simulink model "PathFollower"  (R2024b)
settings: Solver=FixedStepAuto  StartTime=0.0  StopTime=inf  FixedStep=controllerParams.Ts  RelTol=1e-3
PreLoadFcn:
  | % Load scenario parameters if not already loaded
  | if ~exist('hostParams', 'var')
  |     hostParams = helperScenarioParams;
  | end
  | 
  | % Load vehicle parameters if not already loaded
  | if ~exist('vehicleParams', 'var')
  |     vehicleParams = helperVehicleParams;
  | end
  | 
  | % Load PathFollower parameters if not already loaded
  | if ~exist('controllerParams', 'var')
  |     controllerParams = helperPathFollowerParams;
  | end
  | 
  | % Set IP addresses to local computer if they are not provided
  | if ~exist('ipAddress', 'var')
  |     ipAddress = helperIPAddresses;
  | end
libraries: slrealtimeiplib x4, slrealtimeutilitieslib x3, slpidlib x2, simulink x2, robotalgslib x1
settings Model: SimulationMode=external  ExtModeBatchMode=on  ExtModeTrigDuration=100000  Creator=smaddina  LastModifiedBy=demo-user2
settings SolverCC: ConcurrentTasks=on  PositivePriorityOrder=on
settings OptimizationCC: BlockReduction=off  OptimizeBlockIOStorage=off  EnhancedBackFolding=on  PassReuseOutputArgsThreshold=0  MaxStackSize=200000  OptimizeBlockOrder=speed  DifferentSizesBufferReuse=on
settings DebuggingCC: TasksWithSamePriorityMsg=none  ParameterTunabilityLossMsg=error
settings HardwareCC: ProdBitPerLong=64  ProdLongLongMode=on  ProdHWDeviceType=Intel->x86-64 (Linux 64)
settings SFSimCC: MATLABDynamicMemAlloc=off
settings RTWCC: Description=Speedgoat Real-Time Target Machine  SystemTargetFile=speedgoat.tlc  TemplateMakefile=slrealtime_default_tmf  Toolchain=Simulink Real-Time Toolchain  BuildConfiguration=Faster Runs  CodeExecutionProfiling=on  TargetLang=C++
settings CodeAppCC: ForceParamTrailComments=on  OperatorAnnotations=on
settings SimulinkRealTimeTargetCC: InstructionSetFMA=off  LogToMDFFile=off

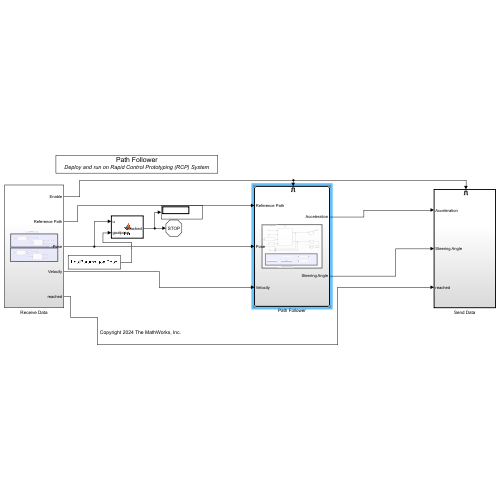
[thumbnail: Simulink's stored preview of the top-level diagram]
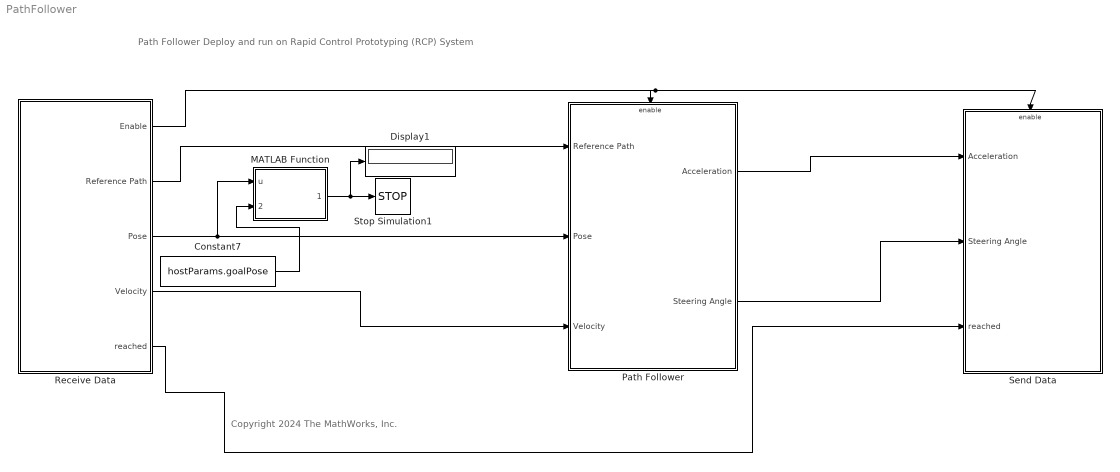
== system PathFollower ==
  note: Path Follower
      | Deploy and run on Rapid Control Prototyping (RCP) System
  note: Copyright 2024 The MathWorks, Inc.
  Constant7 : Constant  Value=hostParams.goalPose
  Display1 : Display
  MATLAB Function : MATLAB Function  TreatAsAtomicUnit=on
  Path Follower : Subsystem
  Receive Data : Subsystem
  Send Data : Subsystem
  Stop Simulation1 : Stop
  wires:
  Receive Data/3(Pose) -> MATLAB Function/1(u), Path Follower/2(Pose)
  Path Follower/1(Acceleration) -> Send Data/1(Acceleration)
  Receive Data/2(Reference Path) -> Path Follower/1(Reference Path)
  Receive Data/4(Velocity) -> Path Follower/3(Velocity)
  Path Follower/2(Steering Angle) -> Send Data/2(Steering Angle)
  Receive Data/1(Enable) -> Send Data/Enable, Path Follower/Enable
  Receive Data/5(reached) -> Send Data/3(reached)
  Constant7/1 -> MATLAB Function/2(goalpose)
  MATLAB Function/1(reached) -> Display1/1, Stop Simulation1/1

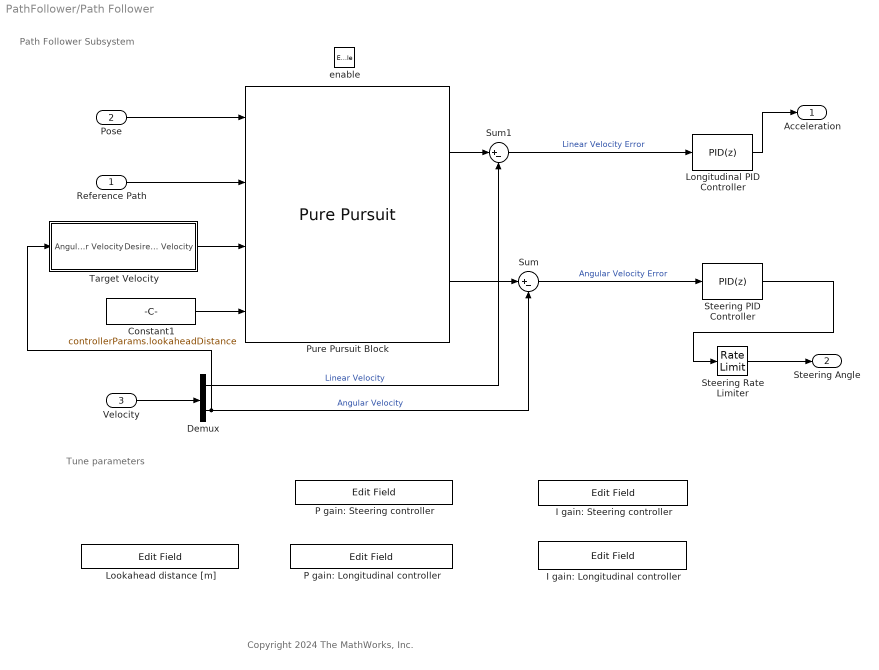
== system PathFollower/Path Follower ==
  note: Path Follower Subsystem
  note: Tune parameters
  note: Copyright 2024 The MathWorks, Inc.
  Reference Path : Inport
  Pose : Inport  Port=2
  Velocity : Inport  Port=3  Interpolate=off
  enable : EnablePort  StatesWhenEnabling=reset
  "       I gain: Longitudinal controller" : EditField  LabelPosition=Hide  ShowInitialText=on  Alignment=Center
  "   I gain: Steering controller" : EditField  LabelPosition=Hide  ShowInitialText=on  Alignment=Center
  Constant1 : Constant  Value=controllerParams.lookaheadDistance
  Demux : Demux  Outputs=2
  Longitudinal PID Controller : slpidlib/PID Controller  Controller=PID  Form=Parallel  TimeDomain=Discrete-time  UseExternalTs=off  SampleTime=-1  IntegratorMethod=Forward Euler  FilterMethod=Forward Euler  ControllerParametersSource=internal  P=controllerParams.accelPGain  I=controllerParams.accelIGain  UseKiTs=off  D=0  UseExternalDerivativeSource=off  N=0  UseFilter=on  TunerSelectOption=Transfer Function Based (PID Tuner App)  InitialConditionSource=internal  InitialConditionForIntegrator=0  InitialConditionForFilter=0  DifferentiatorICPrevScaledInput=0  ExternalReset=none  TrackingMode=off  Kt=1  LimitOutput=on  SatLimitsSource=internal  UpperSaturationLimit=vehicleParams.maxAcceleration  LowerSaturationLimit=vehicleParams.maxDeceleration  LinearizeAsGain=on  AntiWindupMode=none  Kb=1  LimitIntegrator=off  UpperIntegratorSaturationLimit=inf  LowerIntegratorSaturationLimit=-inf  POutMin=[]  POutMax=[]  IOutMin=[]  IOutMax=[]  DOutMin=[]  DOutMax=[]  NOutMin=[]  NOutMax=[]  SumOutMin=[]  SumOutMax=[]  SaturationOutMin=[]  SaturationOutMax=[]  PParamMin=[]  PParamMax=[]  IParamMin=[]  IParamMax=[]  DParamMin=[]  DParamMax=[]  NParamMin=[]  NParamMax=[]  KbParamMin=[]  KbParamMax=[]  KtParamMin=[]  KtParamMax=[]  KbOutMin=[]  KbOutMax=[]  KtOutMin=[]  KtOutMax=[]  IntegratorOutMin=[]  IntegratorOutMax=[]  FilterOutMin=[]  FilterOutMax=[]  SumI1OutMin=[]  SumI1OutMax=[]  SumI2OutMin=[]  SumI2OutMax=[]  SumI3OutMin=[]  SumI3OutMax=[]  SumI4OutMin=[]  SumI4OutMax=[]  SumDOutMin=[]  SumDOutMax=[]  DifferentiatorOutMin=[]  DifferentiatorOutMax=[]  FilterDiffOutCoefMin=[]  FilterDiffOutCoefMax=[]  ReciprocalOutMin=[]  ReciprocalOutMax=[]  SumDenOutMin=[]  SumDenOutMax=[]  SumNumOutMin=[]  SumNumOutMax=[]  DivideOutMin=[]  DivideOutMax=[]  UdiffTsProdOutMin=[]  UdiffTsProdOutMax=[]  NTsProdOutMin=[]  NTsProdOutMax=[]  UintegralTsProdOutMin=[]  UintegralTsProdOutMax=[]  UngainTsProdOutMin=[]  UngainTsProdOutMax=[]  ClampingZeroOutDataTypeStr=Inherit: Inherit via back propagation  ClampingZeroOutMin=[]  ClampingZeroOutMax=[]  FilterDenConstantOutDataTypeStr=Inherit: Inherit via back propagation  FilterDenConstantOutMin=[]  FilterDenConstantOutMax=[]  PCopyOutDataTypeStr=Inherit: Inherit via back propagation  PCopyOutMin=[]  PCopyOutMax=[]  NCopyOutDataTypeStr=Inherit: Inherit via back propagation  NCopyOutMin=[]  NCopyOutMax=[]  IntegratorContinuousStateAttributes=''  IntegratorStateMustResolveToSignalObject=off  IntegratorRTWStateStorageClass=Auto  FilterContinuousStateAttributes=''  FilterStateMustResolveToSignalObject=off  FilterRTWStateStorageClass=Auto  ParallelPVariant=InternalParameters  IdealPVariant=Disabled  IVariant=InternalParameters  DVariant=InternalParameters  IntegratorVariant=Discrete  SatVariant=Enabled  AWVariant=Passthrough  PCopyVariant=Disabled  TRVariant=Disabled  FdbkBlocksVariant=Forward  IdealPFdbkVariant=Disabled  SatFdbkVariant=Disabled  DerivativeFilterVariant=ForwardEulerFilter  NVariant=InternalParameters  NCopyVariant=Disabled  FilterICVariant=InternalICsFilter  IntegratorICVariant=InternalICs  ExternalResetVariant=Disabled  TRSumVariant=Passthrough  SumFdbkVariant=Disabled  SumVariant=Sum_PID  TsampFilterVariant=InternalTs  TsampNgainVariant=Passthrough  TsampIntegralVariant=Disabled_SignalSpec  ExternalSaturationOutDataTypeStr=Inherit: Same as second input  DerivativeSourceVariant=ErrorSignal  PreIntVariant=InternalPreInt
  Lookahead distance [m] : EditField  LabelPosition=Hide  ShowInitialText=on  Alignment=Center
  P gain: Longitudinal controller : EditField  LabelPosition=Hide  ShowInitialText=on  Alignment=Center
  P gain: Steering controller : EditField  LabelPosition=Hide  ShowInitialText=on  Alignment=Center
  Pure Pursuit Block : robotalgslib/Pure Pursuit  DesiredLinearVelocityPort=on  DesiredLinearVelocity=5  MaxAngularVelocity=vehicleParams.maxAngularVelocity  LookaheadDistancePort=on  LookaheadDistance=5  TargetDirPort=off  SimulateUsing=Interpreted execution
  Steering Rate Limiter : RateLimiter  RisingSlewLimit=vehicleParams.maxSteeringAngleRate  FallingSlewLimit=-vehicleParams.maxSteeringAngleRate  SampleTimeMode=inherited
  Steering PID Controller : slpidlib/PID Controller  Controller=PID  Form=Parallel  TimeDomain=Discrete-time  UseExternalTs=off  SampleTime=-1  IntegratorMethod=Forward Euler  FilterMethod=Forward Euler  ControllerParametersSource=internal  P=controllerParams.steeringPGain  I=controllerParams.steeringIGain  UseKiTs=off  D=0  UseExternalDerivativeSource=off  N=0  UseFilter=on  TunerSelectOption=Transfer Function Based (PID Tuner App)  InitialConditionSource=internal  InitialConditionForIntegrator=0  InitialConditionForFilter=0  DifferentiatorICPrevScaledInput=0  ExternalReset=none  TrackingMode=off  Kt=1  LimitOutput=on  SatLimitsSource=internal  UpperSaturationLimit=vehicleParams.maxSteeringAngleRate  LowerSaturationLimit=-vehicleParams.maxSteeringAngleRate  LinearizeAsGain=on  AntiWindupMode=none  Kb=1  LimitIntegrator=off  UpperIntegratorSaturationLimit=inf  LowerIntegratorSaturationLimit=-inf  POutMin=[]  POutMax=[]  IOutMin=[]  IOutMax=[]  DOutMin=[]  DOutMax=[]  NOutMin=[]  NOutMax=[]  SumOutMin=[]  SumOutMax=[]  SaturationOutMin=[]  SaturationOutMax=[]  PParamMin=[]  PParamMax=[]  IParamMin=[]  IParamMax=[]  DParamMin=[]  DParamMax=[]  NParamMin=[]  NParamMax=[]  KbParamMin=[]  KbParamMax=[]  KtParamMin=[]  KtParamMax=[]  KbOutMin=[]  KbOutMax=[]  KtOutMin=[]  KtOutMax=[]  IntegratorOutMin=[]  IntegratorOutMax=[]  FilterOutMin=[]  FilterOutMax=[]  SumI1OutMin=[]  SumI1OutMax=[]  SumI2OutMin=[]  SumI2OutMax=[]  SumI3OutMin=[]  SumI3OutMax=[]  SumI4OutMin=[]  SumI4OutMax=[]  SumDOutMin=[]  SumDOutMax=[]  DifferentiatorOutMin=[]  DifferentiatorOutMax=[]  FilterDiffOutCoefMin=[]  FilterDiffOutCoefMax=[]  ReciprocalOutMin=[]  ReciprocalOutMax=[]  SumDenOutMin=[]  SumDenOutMax=[]  SumNumOutMin=[]  SumNumOutMax=[]  DivideOutMin=[]  DivideOutMax=[]  UdiffTsProdOutMin=[]  UdiffTsProdOutMax=[]  NTsProdOutMin=[]  NTsProdOutMax=[]  UintegralTsProdOutMin=[]  UintegralTsProdOutMax=[]  UngainTsProdOutMin=[]  UngainTsProdOutMax=[]  ClampingZeroOutDataTypeStr=Inherit: Inherit via back propagation  ClampingZeroOutMin=[]  ClampingZeroOutMax=[]  FilterDenConstantOutDataTypeStr=Inherit: Inherit via back propagation  FilterDenConstantOutMin=[]  FilterDenConstantOutMax=[]  PCopyOutDataTypeStr=Inherit: Inherit via back propagation  PCopyOutMin=[]  PCopyOutMax=[]  NCopyOutDataTypeStr=Inherit: Inherit via back propagation  NCopyOutMin=[]  NCopyOutMax=[]  IntegratorContinuousStateAttributes=''  IntegratorStateMustResolveToSignalObject=off  IntegratorRTWStateStorageClass=Auto  FilterContinuousStateAttributes=''  FilterStateMustResolveToSignalObject=off  FilterRTWStateStorageClass=Auto  ParallelPVariant=InternalParameters  IdealPVariant=Disabled  IVariant=InternalParameters  DVariant=InternalParameters  IntegratorVariant=Discrete  SatVariant=Enabled  AWVariant=Passthrough  PCopyVariant=Disabled  TRVariant=Disabled  FdbkBlocksVariant=Forward  IdealPFdbkVariant=Disabled  SatFdbkVariant=Disabled  DerivativeFilterVariant=ForwardEulerFilter  NVariant=InternalParameters  NCopyVariant=Disabled  FilterICVariant=InternalICsFilter  IntegratorICVariant=InternalICs  ExternalResetVariant=Disabled  TRSumVariant=Passthrough  SumFdbkVariant=Disabled  SumVariant=Sum_PID  TsampFilterVariant=InternalTs  TsampNgainVariant=Passthrough  TsampIntegralVariant=Disabled_SignalSpec  ExternalSaturationOutDataTypeStr=Inherit: Same as second input  DerivativeSourceVariant=ErrorSignal  PreIntVariant=InternalPreInt
  Sum : Sum  Inputs=|+-
  Sum1 : Sum  Inputs=|+-
  Target Velocity : Subsystem
  Acceleration : Outport
  Steering Angle : Outport  Port=2
  wires:
  Sum/1 -> Steering PID Controller/1  "Angular Velocity Error"
  Velocity/1 -> Demux/1
  Pure Pursuit Block/2 -> Sum/1
  Reference Path/1 -> Pure Pursuit Block/2
  Pose/1 -> Pure Pursuit Block/1
  Demux/1 -> Sum1/2  "Linear Velocity"
  Demux/2 -> Sum/2, Target Velocity/1(Angular Velocity)  "Angular Velocity"
  Steering Rate Limiter/1 -> Steering Angle/1
  Sum1/1 -> Longitudinal PID Controller/1  "Linear Velocity Error"
  Longitudinal PID Controller/1 -> Acceleration/1
  Pure Pursuit Block/1 -> Sum1/1
  Constant1/1 -> Pure Pursuit Block/4
  Target Velocity/1(Desired Velocity) -> Pure Pursuit Block/3
  Steering PID Controller/1 -> Steering Rate Limiter/1

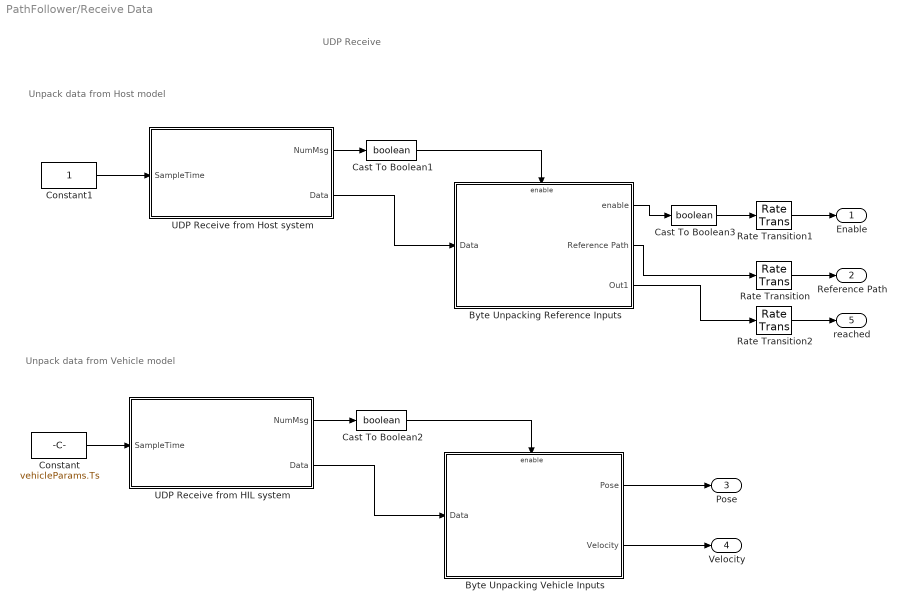
== system PathFollower/Receive Data ==
  note: Unpack data from Vehicle model
  note: Unpack data from Host model
  note: UDP Receive
  Byte Unpacking Reference Inputs : Subsystem  TreatAsAtomicUnit=on
  Byte Unpacking Vehicle Inputs : Subsystem  TreatAsAtomicUnit=on
  Cast To Boolean1 : DataTypeConversion  OutDataTypeStr=boolean  SaturateOnIntegerOverflow=off  RndMeth=Floor
  Cast To Boolean2 : DataTypeConversion  OutDataTypeStr=boolean  SaturateOnIntegerOverflow=off  RndMeth=Floor
  Cast To Boolean3 : DataTypeConversion  OutDataTypeStr=boolean  SaturateOnIntegerOverflow=off  RndMeth=Floor
  Constant : Constant  Value=vehicleParams.Ts  SampleTime=vehicleParams.Ts
  Constant1 : Constant  SampleTime=1
  Rate Transition : RateTransition
  Rate Transition1 : RateTransition
  Rate Transition2 : RateTransition
  UDP Receive from HIL system : Subsystem  TreatAsAtomicUnit=on
  UDP Receive from Host system : Subsystem  TreatAsAtomicUnit=on
  Enable : Outport
  Reference Path : Outport  Port=2
  Pose : Outport  Port=3
  Velocity : Outport  Port=4
  reached : Outport  Port=5
  wires:
  UDP Receive from Host system/1(NumMsg) -> Cast To Boolean1/1
  Cast To Boolean1/1 -> Byte Unpacking Reference Inputs/Enable
  UDP Receive from Host system/2(Data) -> Byte Unpacking Reference Inputs/1(Data)
  Constant1/1 -> UDP Receive from Host system/1(SampleTime)
  Constant/1 -> UDP Receive from HIL system/1(SampleTime)
  Cast To Boolean2/1 -> Byte Unpacking Vehicle Inputs/Enable
  UDP Receive from HIL system/2(Data) -> Byte Unpacking Vehicle Inputs/1(Data)
  UDP Receive from HIL system/1(NumMsg) -> Cast To Boolean2/1
  Byte Unpacking Vehicle Inputs/1(Pose) -> Pose/1
  Byte Unpacking Vehicle Inputs/2(Velocity) -> Velocity/1
  Byte Unpacking Reference Inputs/1(enable) -> Cast To Boolean3/1
  Rate Transition/1 -> Reference Path/1
  Rate Transition1/1 -> Enable/1
  Cast To Boolean3/1 -> Rate Transition1/1
  Byte Unpacking Reference Inputs/2(Reference Path) -> Rate Transition/1
  Byte Unpacking Reference Inputs/3(Out1) -> Rate Transition2/1
  Rate Transition2/1 -> reached/1

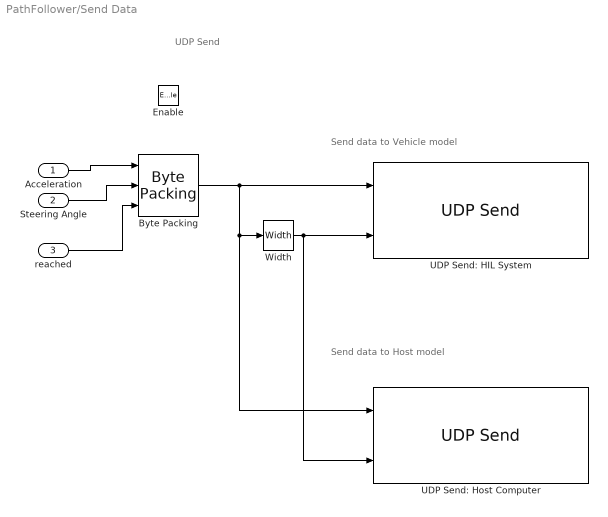
== system PathFollower/Send Data ==
  note: UDP Send
  note: Send data to Host model
  note: Send data to Vehicle model
  Acceleration : Inport
  Steering Angle : Inport  Port=2
  reached : Inport  Port=3
  Enable : EnablePort
  Byte Packing : slrealtimeutilitieslib/Byte Packing  MaskPackedDataType=uint8  MaskUnpackedDataTypes={'double', 'double', 'boolean'}  MaskAlignment=1
  UDP Send: HIL System : slrealtimeiplib/UDP Send  useHostTargetConn=on  toAddress=ipAddress.hilSystem  toPort=8003  sampleTime=-1  enableMessage=off
  UDP Send: Host Computer : slrealtimeiplib/UDP Send  useHostTargetConn=on  toAddress=ipAddress.hostSystem  toPort=8004  sampleTime=-1  enableMessage=off
  Width : Width
  wires:
  Steering Angle/1 -> Byte Packing/2
  Byte Packing/1 -> UDP Send: Host Computer/1, Width/1, UDP Send: HIL System/1
  Width/1 -> UDP Send: Host Computer/2, UDP Send: HIL System/2
  Acceleration/1 -> Byte Packing/1
  reached/1 -> Byte Packing/3

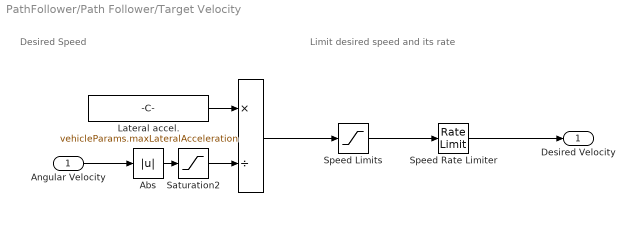
== system PathFollower/Path Follower/Target Velocity ==
  note: Limit desired speed and its rate
  note: Desired Speed
  Angular Velocity : Inport
  " " : Product  Inputs=*/
  Abs : Abs  SaturateOnIntegerOverflow=off
  Lateral accel. : Constant  Value=vehicleParams.maxLateralAcceleration  SampleTime=-1
  Saturation2 : Saturate  UpperLimit=inf  LowerLimit=pi/180
  Speed Rate Limiter : RateLimiter  RisingSlewLimit=vehicleParams.maxAcceleration  FallingSlewLimit=vehicleParams.maxDeceleration  SampleTimeMode=inherited
  Speed Limits : Saturate  UpperLimit=controllerParams.desiredVelocity  LowerLimit=0
  Desired Velocity : Outport
  wires:
  Abs/1 -> Saturation2/1
  Saturation2/1 -> " "/2
  " "/1 -> Speed Limits/1
  Speed Limits/1 -> Speed Rate Limiter/1
  Angular Velocity/1 -> Abs/1
  Lateral accel./1 -> " "/1
  Speed Rate Limiter/1 -> Desired Velocity/1

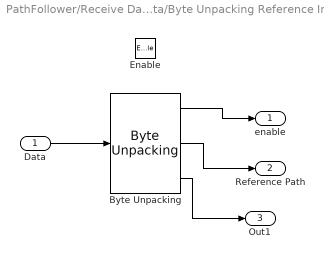
== system PathFollower/Receive Data/Byte Unpacking Reference Inputs ==
  Data : Inport
  Enable : EnablePort
  Byte Unpacking : slrealtimeutilitieslib/Byte Unpacking  MaskUnpackedDataTypes={'double', 'double', 'boolean'}  MaskUnpackedDataSizes={[1], [hostParams.referencePathSize, 2],[1]}  MaskAlignment=1
  enable : Outport
  Reference Path : Outport  Port=2
  Out1 : Outport  Port=3
  wires:
  Data/1 -> Byte Unpacking/1
  Byte Unpacking/1 -> enable/1
  Byte Unpacking/2 -> Reference Path/1
  Byte Unpacking/3 -> Out1/1

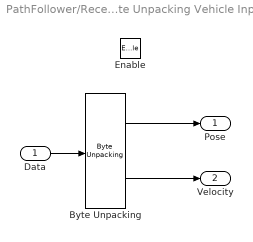
== system PathFollower/Receive Data/Byte Unpacking Vehicle Inputs ==
  Data : Inport
  Enable : EnablePort
  Byte Unpacking : slrealtimeutilitieslib/Byte Unpacking  MaskUnpackedDataTypes={'double', 'double'}  MaskUnpackedDataSizes={[1,3], [1,2]}  MaskAlignment=1
  Pose : Outport
  Velocity : Outport  Port=2
  wires:
  Data/1 -> Byte Unpacking/1
  Byte Unpacking/1 -> Pose/1
  Byte Unpacking/2 -> Velocity/1

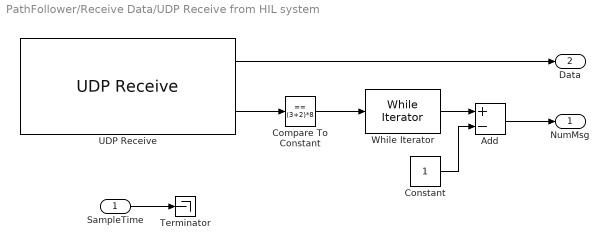
== system PathFollower/Receive Data/UDP Receive from HIL system ==
  SampleTime : Inport
  Add : Sum  Inputs=+-
  Compare To Constant : simulink/Logic and Bit Operations/Compare To Constant  relop===  const=(3+2)*8  OutDataTypeStr=boolean
  Constant : Constant
  Terminator : Terminator
  UDP Receive : slrealtimeiplib/UDP Receive  useHostTargetConn=on  ipAddress=10.10.10.15  localPort=8002  rcvWidth=(3+2)*8  rcvFmAny=on  fmAddress='10.10.10.10'  sampleTime=-1  enableMessage=off  maxPackets=1
  While Iterator : WhileIterator  WhileBlockType=do-while  ShowIterationPort=on
  NumMsg : Outport
  Data : Outport  Port=2
  wires:
  Compare To Constant/1 -> While Iterator/1
  UDP Receive/1 -> Data/1
  UDP Receive/2 -> Compare To Constant/1
  Add/1 -> NumMsg/1
  While Iterator/1 -> Add/1
  Constant/1 -> Add/2
  SampleTime/1 -> Terminator/1

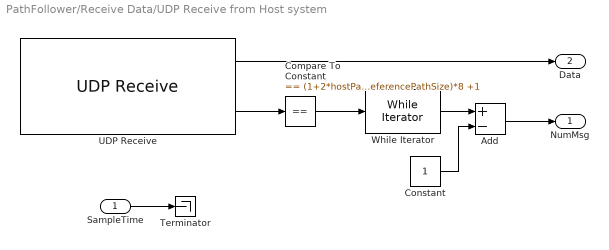
== system PathFollower/Receive Data/UDP Receive from Host system ==
  SampleTime : Inport
  Add : Sum  Inputs=+-
  Compare To Constant : simulink/Logic and Bit Operations/Compare To Constant  relop===  const=(1+2*hostParams.referencePathSize)*8 +1  OutDataTypeStr=boolean
  Constant : Constant
  Terminator : Terminator
  UDP Receive : slrealtimeiplib/UDP Receive  useHostTargetConn=on  ipAddress=10.10.10.15  localPort=8001  rcvWidth=(1+2*hostParams.referencePathSize)*8+1  rcvFmAny=on  fmAddress='10.10.10.10'  sampleTime=-1  enableMessage=off  maxPackets=1
  While Iterator : WhileIterator  WhileBlockType=do-while  ShowIterationPort=on
  NumMsg : Outport
  Data : Outport  Port=2
  wires:
  Compare To Constant/1 -> While Iterator/1
  UDP Receive/1 -> Data/1
  UDP Receive/2 -> Compare To Constant/1
  Add/1 -> NumMsg/1
  While Iterator/1 -> Add/1
  Constant/1 -> Add/2
  SampleTime/1 -> Terminator/1

== matlab function PathFollower/MATLAB Function ==
  data: u input; reached output; goalpose input
function reached = fcn(u, goalpose)
%#codegen

distance = sqrt((u([1])-goalpose([1]))^2 +(u([2])-goalpose([2]))^2 );
if distance<=5
    reached = true;
else

   reached = false;
end
% velgain = 1;
% pose = u;
end
